simulink model "test_EE_ver02"  (R2017a)
settings: Solver=VariableStepAuto  StartTime=0.0  StopTime=inf  RelTol=1e-3
undefined symbols (not defined in the file): serial
libraries: instrumentlib x3, sldrtlib x1, simulink x1
settings Model: Creator=F.Takuya_ASUS  LastModifiedBy=tomato

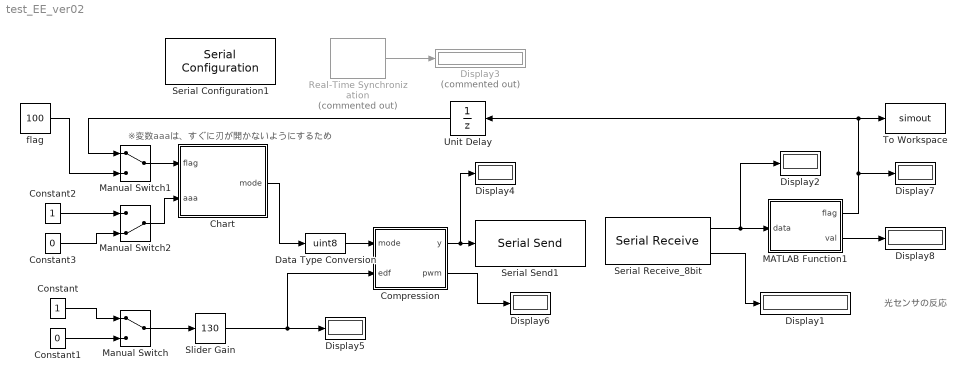
== system test_EE_ver02 ==
  note: 光センサの反応
  note: ※変数aaaは、すぐに刃が開かないようにするため
  Chart : Stateflow chart  TreatAsAtomicUnit=on
  Compression : MATLAB Function  TreatAsAtomicUnit=on
  Constant : Constant  SampleTime=0.1
  Constant1 : Constant  Value=0  SampleTime=0.1
  Constant2 : Constant  SampleTime=0.1
  Constant3 : Constant  Value=0  SampleTime=0.1
  Data Type Conversion : DataTypeConversion  OutDataTypeStr=uint8
  Display{1..2,4..8} (7 alike) : Display
  Display3 : Display  Commented=on
  MATLAB Function1 : MATLAB Function  TreatAsAtomicUnit=on
  Manual Switch : ManualSwitch
  Manual Switch1 : ManualSwitch
  Manual Switch2 : ManualSwitch  CurrentSetting=0
  Real-Time Synchronization : sldrtlib/Real-Time Synchronization  Commented=on  SampleTime=0.1  MaxMissedTicks=inf  ShowMissedTicks=on  YieldWhenWaiting=off
  Serial Configuration1 : instrumentlib/Serial Configuration  Priority=-200000  ComPortMenu=COM3  ComPort=COM3  ObjConstructor=serial('COM3');  BaudRate=115200  DataBits=8  Parity=none  StopBits=1  FlowControl=none  Timeout=10  ByteOrder=LittleEndian
  Serial Receive_8bit : instrumentlib/Serial Receive  ComPortMenu=COM3  ComPort=COM3  ObjConstructor=serial('COM3');  Terminator=<none>  DataSize=1  DataType=uint8  EnableBlockingMode=off  ActionDataUnavailable=Output last received value  CustomValue=0  SampleTime=0.1
  Serial Send1 : instrumentlib/Serial Send  ComPortMenu=COM3  ComPort=COM3  ObjConstructor=serial('COM3');  Terminator=<none>  EnableBlockingMode=off
  Slider Gain : simulink/Math Operations/Slider Gain  gain=130  low=0  high=200
  To Workspace : ToWorkspace  VariableName=simout  SaveFormat=Timeseries  SampleTime=-1
  Unit Delay : UnitDelay  SampleTime=-1
  flag : Constant  Value=100  OutDataTypeStr=uint8  SampleTime=0.1
  wires:
  Slider Gain/1 -> Compression/2(edf), Display5/1
  Compression/2(pwm) -> Display6/1
  MATLAB Function1/2(val) -> Display8/1
  Serial Receive_8bit/1 -> Display2/1, MATLAB Function1/1(data)
  Compression/1(y) -> Display4/1, Serial Send1/1
  MATLAB Function1/1(flag) -> To Workspace/1, Unit Delay/1, Display7/1
  Serial Receive_8bit/2 -> Display1/1
  Constant/1 -> Manual Switch/1
  flag/1 -> Manual Switch1/2
  Manual Switch/1 -> Slider Gain/1
  Constant1/1 -> Manual Switch/2
  Real-Time Synchronization/1 -> Display3/1
  Chart/1(mode) -> Data Type Conversion/1
  Manual Switch1/1 -> Chart/1(flag)
  Unit Delay/1 -> Manual Switch1/1
  Data Type Conversion/1 -> Compression/1(mode)
  Manual Switch2/1 -> Chart/2(aaa)
  Constant2/1 -> Manual Switch2/1
  Constant3/1 -> Manual Switch2/2

== matlab function test_EE_ver02/MATLAB Function1 ==
  data: flag output; data input; val output
function [flag,val] = fcn(data)

% 入力(data)を右に5bitシフトして、上位3bitを取り出す
flag = uint8(bitshift(data,-5));

% 入力(data)と31(00011111)のAND演算をして、下位5bitを取り出す
a = double(bitand(data, 31));

val = double(a * 10 + 800);

== matlab function test_EE_ver02/Compression ==
  data: mode input; edf input; y output; pwm output
function [y,pwm] = fcn(mode, edf)

if mode < 0
    mode = uint8(0);
elseif mode > 7
    mode = uint8(7);
end

if edf > 200
    edf = 200;
end

pwm = uint8(floor(edf / 10));

y = bitshift(mode,5) + pwm;

== stateflow chart test_EE_ver02/Chart ==
  state m03/
    % 切断2
    entry:
    mode=3;
  state m0/
    % 待機
    entry:
    mode=0;
  state m04/
    % 把持
    entry:
    mode=4;
  state m01/
    % 吸引
    entry:
    mode=1;
  state m02/
    % 切断1
    entry:
    mode=2;
  m04 -> m0 [order 2] : [flag == 0]
  (default) -> m0
  m01 -> m0 [commented out] : after(10, sec)
  m02 -> m03 : [(flag == 6 && aaa == 1) ]%|| after(5,sec)]
  m0 -> m01 : [flag == 100]
  m03 -> m04 : %after(2,sec)%
      | [flag == 7]
  m01 -> m02 : [flag == 5]
  m04 -> m04 [order 1] : [flag == 4]
  data: flag input; mode output; aaa input
